simulink model "modello_Sabas_friend"  (R2020b)
settings: Solver=FixedStepAuto  StartTime=0.0  StopTime=5000  MinStep=0.009999  RelTol=1e-3
undefined symbols (not defined in the file or in its folder): Omega_0, omega_0
libraries: simulink x3, vrlib x1, aerolibatmos2 x1, sharedutil x1, aerolibgravity2 x1, sharedtransform x1
settings Model: Creator=Qmars  LastModifiedBy=Alessia

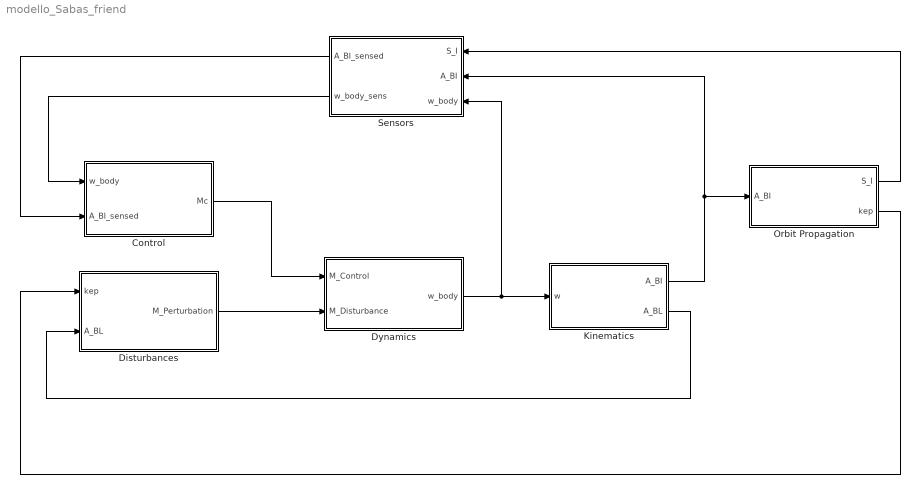
== system modello_Sabas_friend ==
  Control : Subsystem  mask{Control_Option=Target Pointing, MagMax=1.19, MagTorq_error=0.005, sample_rate_Mag=10, Irw=1e-5, maxRPM=8000, RPM_acc=5, sample_rate_RW=1, maxRPMrate=100, K_Det_x=-0.005*0.1585, K_Det_y=-0.005*0.0921, K_Det_z=-0.005*0.0866, Kp_Target_Pointing_x=-0.0027*0.1585, Kp_Target_Pointing_y=-0.0027*0.0921, Kp_Target_Pointing_z=-0.0027*0.0866, Kd_Target_Pointing_x=-0.104*0.1585, Kd_Target_Pointing_y=-0.104*0.0921, Kd_Target_Pointing_z=-0.104*0.0866}
      mask prompts: Control_Option "Choose your desired control strategy:"; MagMax "Max Magnetic Dipole (A.m^2)"; MagTorq_error "Dipole Error (A.m^2)"; sample_rate_Mag "Sample Rate [Hz]"; Irw "Moment of Inertia [kg.m^2]"; maxRPM "Max RPM"; RPM_acc "RPM Accuracy"; sample_rate_RW "Sample Rate [Hz]"; maxRPMrate "Max RPM Rate"
      mask TypeOptions Control_Option: No Control | Detumbling | Target Pointing
      mask DialogControl Container6 Prompt: Control Strategy
      mask DialogControl Container7 Prompt: Magnetorqure
      mask DialogControl Container8 Prompt: Reaction Wheels
      mask DialogControl Container10 Prompt: Detumbling Parameters
      mask DialogControl Container11 Prompt: Target Pointing
      mask Display: disp("Control")
  Disturbances : Subsystem  mask{rho_s_main=0.5, rho_d_main=0.1, rho_s_SP=0, rho_d_SP=0, C_D_main=2.2, C_D_SP=2.2}
      mask prompts: rho_s_main "Specular Reflection Coefficient"; rho_d_main "Diffusion Coefficient"; rho_s_SP "Specular Reflection Coefficient"; rho_d_SP "Diffusion Coefficient"; C_D_main "Drag Coefficient"; C_D_SP "Drag Coefficient"
      mask DialogControl Container4 Prompt: Radiation Constants
      mask DialogControl Container5 Prompt: Main Body
      mask DialogControl Container6 Prompt: Solar Panels
      mask DialogControl Container7 Prompt: Aerodynamics
      mask DialogControl Container10 Prompt: Main Body
      mask DialogControl Container11 Prompt: Solar Panels
      mask Display: disp("Disturbances")
  Dynamics : Subsystem  mask{m_main=9, b=0.1, d=0.3, a=0.2, m_SP=0.6, c=0.2, w_x_0=0.5, w_y_0=0.5, w_z_0=0.5}
      mask prompts: m_main "Mass [kg]"; b "Length in the X direction [m]"; d "Length in the Y direction [m]"; a "Length in the Z direction [m]"; m_SP "Mass [kg]"; c "Width in the Z direction [m]"; w_x_0 "Initial angular velocity in the X direction [deg/sec]"; w_y_0 "Initial angular velocity in the Y direction [deg/sec]"; w_z_0 "Initial angular velocity in the Z direction [deg/sec]"
      mask DialogControl Container4 Prompt: Satellite Characteristics
      mask DialogControl Container5 Prompt: Main Body
      mask DialogControl Container6 Prompt: Solar Panels
      mask DialogControl Container7 Prompt: Initial Conditions
      mask Display: disp("Dynamics")
  Kinematics : Subsystem  mask{theta_1_0=10, theta_2_0=10, theta_3_0=10}
      mask prompts: theta_1_0 "First Angle [deg]"; theta_2_0 "Second Angle [deg]"; theta_3_0 "Third Angle [deg]"
      mask DialogControl Container4 Prompt: Initial Conditions
      mask Display: disp("Kinematics")
  Orbit Propagation : Subsystem  mask{a_orbit=7092, e=0.0641568, i=98, omega=0, theta_0=270, Year=2021, Month=3, Day=21, Hour=12, Minute=0, Second=0}
      mask prompts: a_orbit "Semi-Major Axis [km]"; e "Eccentricity"; i "Inclination [deg]"; omega "Angular Position of the Perigee [deg]"; theta_0 "Initial Satellite Position [deg]"; Month "Month [number]"
      mask DialogControl Container4 Prompt: Orbit
      mask DialogControl Container5 Prompt: Time
      mask Display: disp("Orbit Propagation")
  Sensors : Subsystem  mask{accuracy_Sun=0.5, sample_rate_Sun=5, accuracy_EH=0.25, sample_rate_EH=1, accuracy_Star=1/360, sample_rate_Star=5, Mag_acc=1, sample_rate_Mag=10, ARW=0.2, RRW=0.3, sample_rate_Gyro=10}
      mask prompts: accuracy_Sun "Accuracy [deg]"; sample_rate_Sun "Sample Rate [Hz]"; accuracy_EH "Accuracy [deg]"; sample_rate_EH "Sample Rate [Hz]"; accuracy_Star "Accuracy [deg]"; sample_rate_Star "Sample Rate [Hz]"; Mag_acc "Accuracy [deg]"; sample_rate_Mag "Sample Rate [Hz]"; ARW "Angular Random Walk(ARW) [deg/hr^0.5]"; RRW "Rate Random Walk(RRW) [deg/hr^1.5]"; sample_rate_Gyro "Sample Rate [Hz]"
      mask DialogControl Container4 Prompt: Attitude Sensors
      mask DialogControl Container7 Prompt: Sun Sensor
      mask DialogControl Container9 Prompt: Earth Horizon Sensor
      mask DialogControl Container10 Prompt: Star Sensor
      mask DialogControl Container14 Prompt: Magnetometer
      mask DialogControl Container11 Prompt: Gyro
      mask Display: disp("Sensors")
  wires:
  Disturbances/1(M_Perturbation) -> Dynamics/2(M_Disturbance)
  Dynamics/1(w_body) -> Sensors/3(w_body), Kinematics/1(w)
  Kinematics/1(A_BI) -> Orbit Propagation/1(A_BI), Sensors/2(A_BI)
  Orbit Propagation/1(S_I) -> Sensors/1(S_I)
  Kinematics/2(A_BL) -> Disturbances/2(A_BL)
  Sensors/2(w_body_sens) -> Control/1(w_body)
  Control/1(Mc) -> Dynamics/1(M_Control)
  Sensors/1(A_BI_sensed) -> Control/2(A_BI_sensed)
  Orbit Propagation/2(kep) -> Disturbances/1(kep)

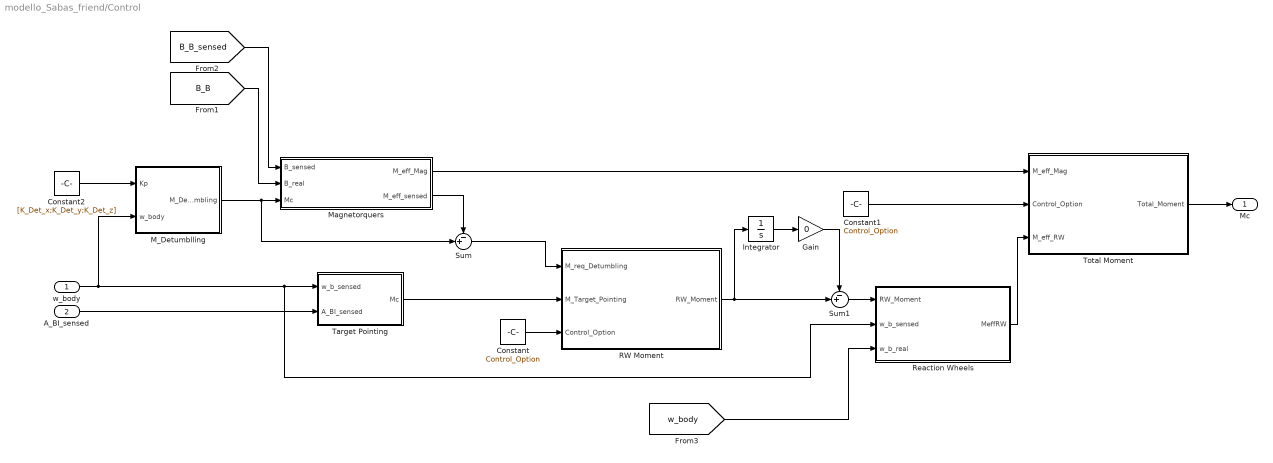
== system modello_Sabas_friend/Control ==
  w_body : Inport
  A_BI_sensed : Inport  Port=2
  Constant : Constant  Value=Control_Option
  Constant1 : Constant  Value=Control_Option
  Constant2 : Constant  Value=[K_Det_x;K_Det_y;K_Det_z]
  Gain : Gain  Gain=0
  Integrator : Integrator
  M_Detumblling : MATLAB Function  TreatAsAtomicUnit=on
  Magnetorquers : Subsystem
  RW Moment : MATLAB Function  TreatAsAtomicUnit=on
  Reaction Wheels : Subsystem
  Sum : Sum  Inputs=-+|
  Sum1 : Sum  Inputs=-+|
  Target Pointing : Subsystem
  Total Moment : MATLAB Function  TreatAsAtomicUnit=on
  Mc : Outport
  wires:
  M_Detumblling/1(M_Detumbling) -> Sum/2, Magnetorquers/3(Mc)
  w_body/1 -> M_Detumblling/2(w_body), Reaction Wheels/2(w_b_sensed), Target Pointing/1(w_b_sensed)
  A_BI_sensed/1 -> Target Pointing/2(A_BI_sensed)
  [B_B] -> Magnetorquers/2(B_real)
  [B_B_sensed] -> Magnetorquers/1(B_sensed)
  Target Pointing/1(Mc) -> RW Moment/2(M_Target_Pointing)
  Magnetorquers/2(M_eff_sensed) -> Sum/1
  Sum/1 -> RW Moment/1(M_req_Detumbling)
  Constant/1 -> RW Moment/3(Control_Option)
  RW Moment/1(RW_Moment) -> Integrator/1, Sum1/2
  [w_body] -> Reaction Wheels/3(w_b_real)
  Constant1/1 -> Total Moment/2(Control_Option)
  Reaction Wheels/1(MeffRW) -> Total Moment/3(M_eff_RW)
  Magnetorquers/1(M_eff_Mag) -> Total Moment/1(M_eff_Mag)
  Total Moment/1(Total_Moment) -> Mc/1
  Constant2/1 -> M_Detumblling/1(Kp)
  Sum1/1 -> Reaction Wheels/1(RW_Moment)
  Integrator/1 -> Gain/1
  Gain/1 -> Sum1/1

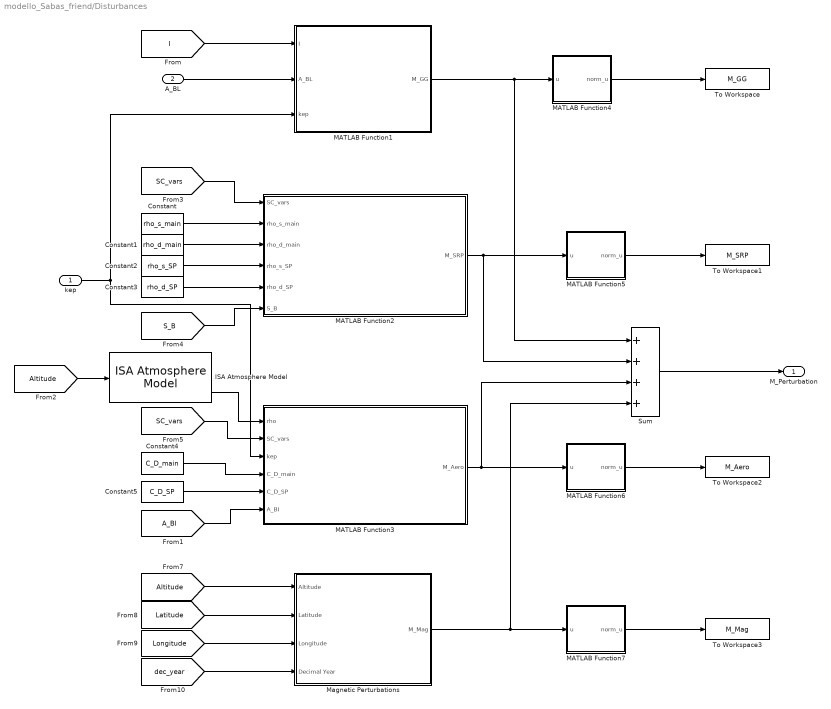
== system modello_Sabas_friend/Disturbances ==
  kep : Inport
  A_BL : Inport  Port=2
  Constant : Constant  Value=rho_s_main
  Constant1 : Constant  Value=rho_d_main
  Constant2 : Constant  Value=rho_s_SP
  Constant3 : Constant  Value=rho_d_SP
  Constant4 : Constant  Value=C_D_main
  Constant5 : Constant  Value=C_D_SP
  ISA Atmosphere Model : aerolibatmos2/ISA Atmosphere Model  custom=off  g=9.80665  gamma=1.4  R=287.0531  L=0.0065  h_trop=11000  h_strat=20000  rho0=1.225  P0=101325  T0=288.15  h0=0
  MATLAB Function1 : MATLAB Function  TreatAsAtomicUnit=on
  MATLAB Function2 : MATLAB Function  TreatAsAtomicUnit=on
  MATLAB Function3 : MATLAB Function  TreatAsAtomicUnit=on
  MATLAB Function4 : MATLAB Function  TreatAsAtomicUnit=on
  MATLAB Function5 : MATLAB Function  TreatAsAtomicUnit=on
  MATLAB Function6 : MATLAB Function  TreatAsAtomicUnit=on
  MATLAB Function7 : MATLAB Function  TreatAsAtomicUnit=on
  Magnetic Perturbations : Subsystem
  Sum : Sum  Inputs=++++
  To Workspace : ToWorkspace  VariableName=M_GG  SaveFormat=Structure With Time  SampleTime=-1
  To Workspace1 : ToWorkspace  VariableName=M_SRP  SaveFormat=Structure With Time  SampleTime=-1
  To Workspace2 : ToWorkspace  VariableName=M_Aero  SaveFormat=Structure With Time  SampleTime=-1
  To Workspace3 : ToWorkspace  VariableName=M_Mag  SaveFormat=Structure With Time  SampleTime=-1
  M_Perturbation : Outport
  wires:
  [dec_year] -> Magnetic Perturbations/4(Decimal Year)
  [I] -> MATLAB Function1/1(I)
  A_BL/1 -> MATLAB Function1/2(A_BL)
  [SC_vars] -> MATLAB Function2/1(SC_vars)
  Constant/1 -> MATLAB Function2/2(rho_s_main)
  [S_B] -> MATLAB Function2/6(S_B)
  Constant1/1 -> MATLAB Function2/3(rho_d_main)
  Constant2/1 -> MATLAB Function2/4(rho_s_SP)
  Constant3/1 -> MATLAB Function2/5(rho_d_SP)
  [SC_vars] -> MATLAB Function3/2(SC_vars)
  kep/1 -> MATLAB Function1/3(kep), MATLAB Function3/3(kep)
  Constant4/1 -> MATLAB Function3/4(C_D_main)
  Constant5/1 -> MATLAB Function3/5(C_D_SP)
  [Latitude] -> Magnetic Perturbations/2(Latitude)
  [Altitude] -> Magnetic Perturbations/1(Altitude)
  [Longitude] -> Magnetic Perturbations/3(Longitude)
  MATLAB Function1/1(M_GG) -> Sum/1, MATLAB Function4/1(u)
  MATLAB Function2/1(M_SRP) -> MATLAB Function5/1(u), Sum/2
  MATLAB Function3/1(M_Aero) -> MATLAB Function6/1(u), Sum/3
  Magnetic Perturbations/1(M_Mag) -> MATLAB Function7/1(u), Sum/4
  Sum/1 -> M_Perturbation/1
  [A_BI] -> MATLAB Function3/6(A_BI)
  ISA Atmosphere Model/4 -> MATLAB Function3/1(rho)
  [Altitude] -> ISA Atmosphere Model/1
  MATLAB Function4/1(norm_u) -> To Workspace/1
  MATLAB Function5/1(norm_u) -> To Workspace1/1
  MATLAB Function6/1(norm_u) -> To Workspace2/1
  MATLAB Function7/1(norm_u) -> To Workspace3/1

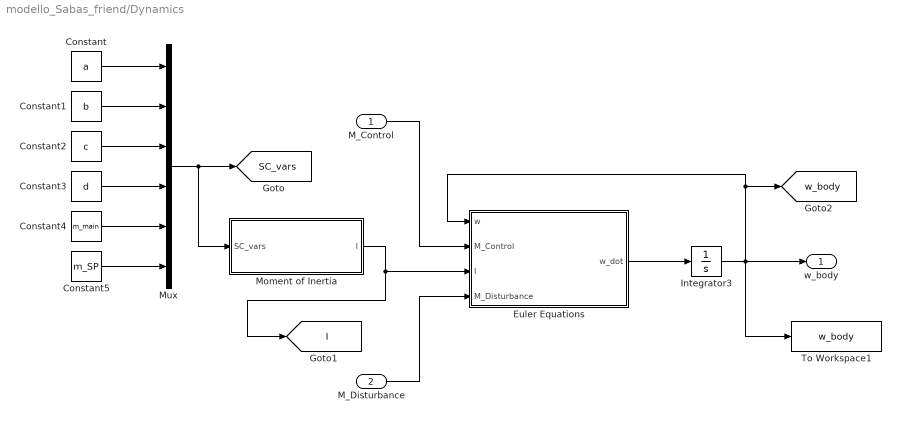
== system modello_Sabas_friend/Dynamics ==
  M_Control : Inport
  M_Disturbance : Inport  Port=2
  Constant : Constant  Value=a
  Constant1 : Constant  Value=b
  Constant2 : Constant  Value=c
  Constant3 : Constant  Value=d
  Constant4 : Constant  Value=m_main
  Constant5 : Constant  Value=m_SP
  Euler Equations : MATLAB Function  TreatAsAtomicUnit=on
  Integrator3 : Integrator  InitialCondition=pi*[w_x_0;w_y_0;w_z_0]/180
  Moment of Inertia : MATLAB Function  TreatAsAtomicUnit=on
  Mux : Mux  Inputs=6
  To Workspace1 : ToWorkspace  VariableName=w_body  SaveFormat=Timeseries  SampleTime=-1
  w_body : Outport
  tag scope: I=global, SC_vars=global, w_body=global
  wires:
  Integrator3/1 -> To Workspace1/1, w_body/1, Euler Equations/1(w), [w_body]
  Moment of Inertia/1(I) -> Euler Equations/3(I), [I]
  Euler Equations/1(w_dot) -> Integrator3/1
  M_Control/1 -> Euler Equations/2(M_Control)
  M_Disturbance/1 -> Euler Equations/4(M_Disturbance)
  Constant/1 -> Mux/1
  Constant1/1 -> Mux/2
  Constant2/1 -> Mux/3
  Constant3/1 -> Mux/4
  Constant4/1 -> Mux/5
  Constant5/1 -> Mux/6
  Mux/1 -> Moment of Inertia/1(SC_vars), [SC_vars]

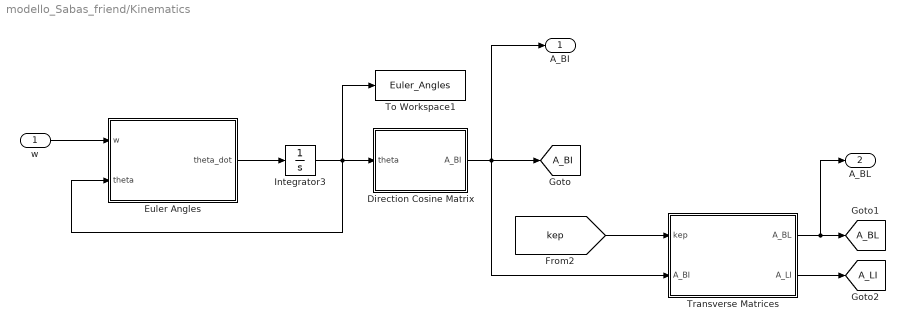
== system modello_Sabas_friend/Kinematics ==
  w : Inport
  Direction Cosine Matrix : MATLAB Function  TreatAsAtomicUnit=on
  Euler Angles : MATLAB Function  TreatAsAtomicUnit=on
  Integrator3 : Integrator  InitialCondition=pi*[theta_1_0;theta_2_0;theta_3_0]/180
  To Workspace1 : ToWorkspace  VariableName=Euler_Angles  SaveFormat=Timeseries  SampleTime=-1
  Transverse Matrices : MATLAB Function  TreatAsAtomicUnit=on
  A_BI : Outport
  A_BL : Outport  Port=2
  tag scope: A_BI=global, A_BL=global, A_LI=global
  wires:
  Integrator3/1 -> To Workspace1/1, Direction Cosine Matrix/1(theta), Euler Angles/2(theta)
  Euler Angles/1(theta_dot) -> Integrator3/1
  w/1 -> Euler Angles/1(w)
  Direction Cosine Matrix/1(A_BI) -> A_BI/1, Transverse Matrices/2(A_BI), [A_BI]
  Transverse Matrices/1(A_BL) -> [A_BL], A_BL/1
  [kep] -> Transverse Matrices/1(kep)
  Transverse Matrices/2(A_LI) -> [A_LI]

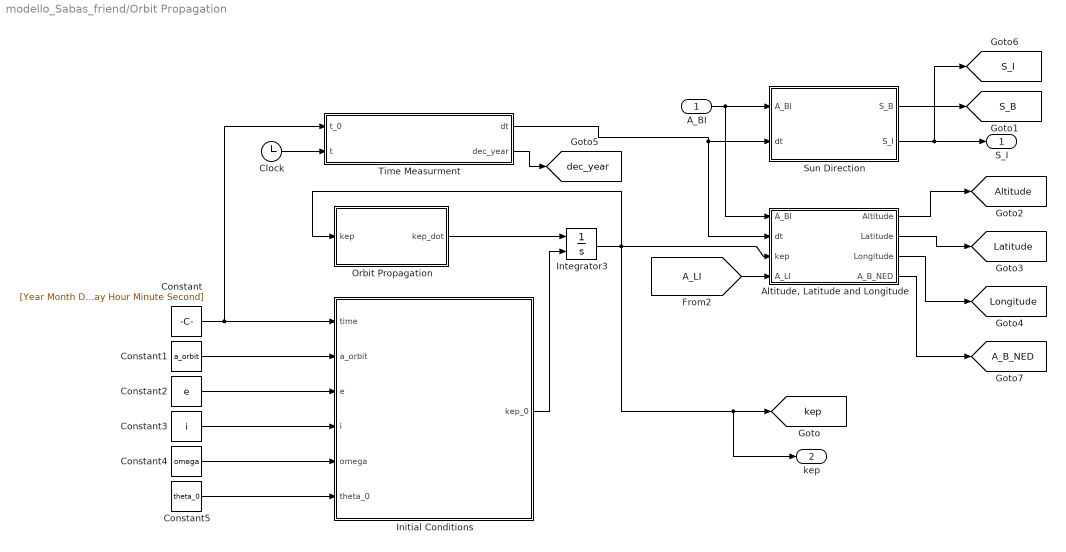
== system modello_Sabas_friend/Orbit Propagation ==
  A_BI : Inport
  "Altitude, Latitude and Longitude" : MATLAB Function  TreatAsAtomicUnit=on
  Clock : Clock
  Constant : Constant  Value=[Year Month Day Hour Minute Second]
  Constant1 : Constant  Value=a_orbit
  Constant2 : Constant  Value=e
  Constant3 : Constant  Value=i
  Constant4 : Constant  Value=omega
  Constant5 : Constant  Value=theta_0
  Initial Conditions : MATLAB Function  TreatAsAtomicUnit=on
  Integrator3 : Integrator  InitialConditionSource=external  InitialCondition=[a_orbit;e;i;Omega_0;omega_0;theta_0]
  Orbit Propagation : MATLAB Function  TreatAsAtomicUnit=on
  Sun Direction : MATLAB Function  TreatAsAtomicUnit=on
  Time Measurment : MATLAB Function  TreatAsAtomicUnit=on
  S_I : Outport
  kep : Outport  Port=2
  tag scope: A_B_NED=global, Altitude=global, Latitude=global, Longitude=global, S_B=global, S_I=global, dec_year=global, kep=global
  wires:
  Orbit Propagation/1(kep_dot) -> Integrator3/1
  Integrator3/1 -> Orbit Propagation/1(kep), "Altitude, Latitude and Longitude"/3(kep), kep/1, [kep]
  A_BI/1 -> "Altitude, Latitude and Longitude"/1(A_BI), Sun Direction/1(A_BI)
  Sun Direction/2(S_I) -> [S_I], S_I/1
  Sun Direction/1(S_B) -> [S_B]
  Initial Conditions/1(kep_0) -> Integrator3/2
  Constant/1 -> Initial Conditions/1(time), Time Measurment/1(t_0)
  Constant1/1 -> Initial Conditions/2(a_orbit)
  Constant2/1 -> Initial Conditions/3(e)
  Constant5/1 -> Initial Conditions/6(theta_0)
  Constant4/1 -> Initial Conditions/5(omega)
  Constant3/1 -> Initial Conditions/4(i)
  Clock/1 -> Time Measurment/2(t)
  Time Measurment/1(dt) -> "Altitude, Latitude and Longitude"/2(dt), Sun Direction/2(dt)
  "Altitude, Latitude and Longitude"/1(Altitude) -> [Altitude]
  "Altitude, Latitude and Longitude"/3(Longitude) -> [Longitude]
  "Altitude, Latitude and Longitude"/2(Latitude) -> [Latitude]
  [A_LI] -> "Altitude, Latitude and Longitude"/4(A_LI)
  Time Measurment/2(dec_year) -> [dec_year]
  "Altitude, Latitude and Longitude"/4(A_B_NED) -> [A_B_NED]

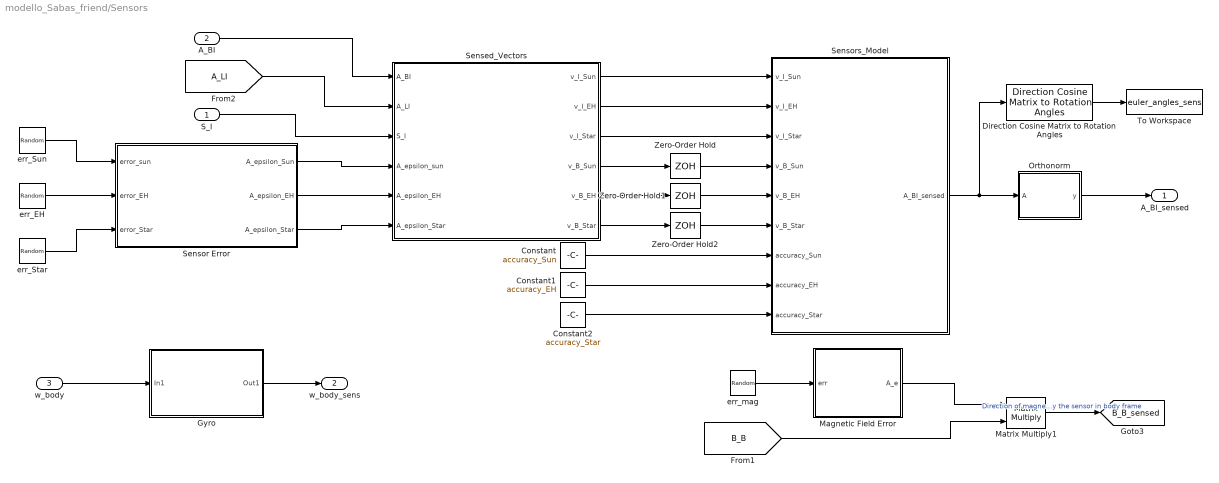
== system modello_Sabas_friend/Sensors ==
  S_I : Inport
  A_BI : Inport  Port=2
  w_body : Inport  Port=3
  Constant : Constant  Value=accuracy_Sun
  Constant1 : Constant  Value=accuracy_EH
  Constant2 : Constant  Value=accuracy_Star
  Direction Cosine Matrix to Rotation Angles : sharedtransform/Direction Cosine Matrix to Rotation Angles  rotationOrder=ZYX  aMode=aMode  action=None  tolerance=eps(2)
      settings: SourceProductBaseCode=AE,PW,DR,MT,UV,VE
  Gyro : Subsystem
  Magnetic Field Error : MATLAB Function  TreatAsAtomicUnit=on
  Matrix Multiply1 : Product  Multiplication=Matrix(*)
  Orthonorm : MATLAB Function  TreatAsAtomicUnit=on
  Sensed_Vectors : MATLAB Function  TreatAsAtomicUnit=on
  Sensor Error : MATLAB Function  TreatAsAtomicUnit=on
  Sensors_Model : MATLAB Function  TreatAsAtomicUnit=on
  To Workspace : ToWorkspace  VariableName=euler_angles_sens  SaveFormat=Timeseries  SampleTime=-1
  Zero-Order Hold : ZeroOrderHold  SampleTime=1/sample_rate_Sun
  Zero-Order Hold1 : ZeroOrderHold  SampleTime=1/sample_rate_EH
  Zero-Order Hold2 : ZeroOrderHold  SampleTime=1/sample_rate_Star
  err_EH : RandomNumber  Variance=(1/4*deg2rad(accuracy_EH*[1 1 1])).^2  Seed=[4 5 6]  SampleTime=1/10
  err_Star : RandomNumber  Variance=(1/4*deg2rad(accuracy_Star*[1 1 1])).^2  Seed=[4 5 6]  SampleTime=1/10
  err_Sun : RandomNumber  Variance=(1/4*deg2rad(accuracy_Sun*[1 1 1])).^2  Seed=[1 2 3]  SampleTime=1/10
  err_mag : RandomNumber  Variance=(1/4*deg2rad(Mag_acc*[1;1;1])).^2  Seed=[1 2 3]  SampleTime=1/sample_rate_Mag
  A_BI_sensed : Outport
  w_body_sens : Outport  Port=2
  tag scope: B_B_sensed=global
  wires:
  err_Sun/1 -> Sensor Error/1(error_sun)
  Constant1/1 -> Sensors_Model/8(accuracy_EH)
  S_I/1 -> Sensed_Vectors/3(S_I)
  err_Star/1 -> Sensor Error/3(error_Star)
  err_EH/1 -> Sensor Error/2(error_EH)
  A_BI/1 -> Sensed_Vectors/1(A_BI)
  Sensors_Model/1(A_BI_sensed) -> Direction Cosine Matrix to Rotation Angles/1, Orthonorm/1(A)
  [A_LI] -> Sensed_Vectors/2(A_LI)
  Constant/1 -> Sensors_Model/7(accuracy_Sun)
  Constant2/1 -> Sensors_Model/9(accuracy_Star)
  Orthonorm/1(y) -> A_BI_sensed/1
  Sensor Error/1(A_epsilon_Sun) -> Sensed_Vectors/4(A_epsilon_sun)
  Sensor Error/2(A_epsilon_EH) -> Sensed_Vectors/5(A_epsilon_EH)
  Sensor Error/3(A_epsilon_Star) -> Sensed_Vectors/6(A_epsilon_Star)
  Sensed_Vectors/2(v_I_EH) -> Sensors_Model/2(v_I_EH)
  Sensed_Vectors/3(v_I_Star) -> Sensors_Model/3(v_I_Star)
  Sensed_Vectors/4(v_B_Sun) -> Zero-Order Hold/1
  Sensed_Vectors/5(v_B_EH) -> Zero-Order Hold1/1
  Sensed_Vectors/6(v_B_Star) -> Zero-Order Hold2/1
  Sensed_Vectors/1(v_I_Sun) -> Sensors_Model/1(v_I_Sun)
  Zero-Order Hold/1 -> Sensors_Model/4(v_B_Sun)
  Zero-Order Hold1/1 -> Sensors_Model/5(v_B_EH)
  Zero-Order Hold2/1 -> Sensors_Model/6(v_B_Star)
  Direction Cosine Matrix to Rotation Angles/1 -> To Workspace/1
  w_body/1 -> Gyro/1(In1)
  Gyro/1(Out1) -> w_body_sens/1
  err_mag/1 -> Magnetic Field Error/1(err)
  Magnetic Field Error/1(A_e) -> Matrix Multiply1/1
  [B_B] -> Matrix Multiply1/2
  Matrix Multiply1/1 -> [B_B_sensed]  "Direction of magnetic field vector determined by the sensor in body frame"

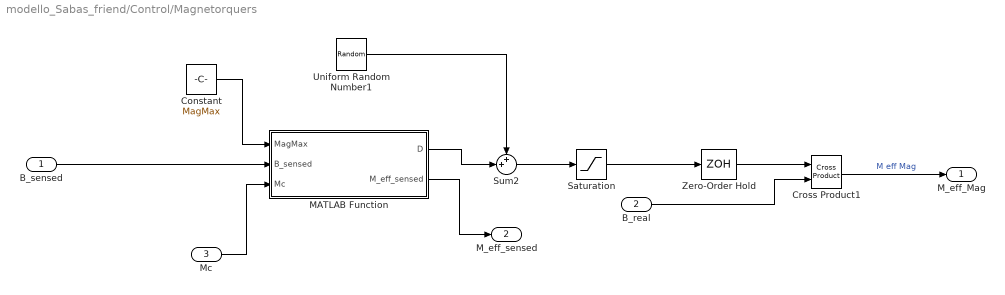
== system modello_Sabas_friend/Control/Magnetorquers ==
  B_sensed : Inport
  B_real : Inport  Port=2
  Mc : Inport  Port=3
  Constant : Constant  Value=MagMax
  Cross Product1 : vrlib/Utilities/Cross Product
  MATLAB Function : MATLAB Function  TreatAsAtomicUnit=on
  Saturation : Saturate  UpperLimit=MagMax  LowerLimit=-MagMax
  Sum2 : Sum  Inputs=++|
  Uniform Random Number1 : UniformRandomNumber  Minimum=-MagTorq_error*[1;1;1]  Maximum=MagTorq_error*[1;1;1]  Seed=456156  SampleTime=1/sample_rate_Mag
  Zero-Order Hold : ZeroOrderHold  SampleTime=1/sample_rate_Mag
  M_eff_Mag : Outport
  M_eff_sensed : Outport  Port=2
  wires:
  B_sensed/1 -> MATLAB Function/2(B_sensed)
  Saturation/1 -> Zero-Order Hold/1
  Cross Product1/1 -> M_eff_Mag/1  "M eff Mag"
  Sum2/1 -> Saturation/1
  Zero-Order Hold/1 -> Cross Product1/1
  Constant/1 -> MATLAB Function/1(MagMax)
  MATLAB Function/1(D) -> Sum2/2
  B_real/1 -> Cross Product1/2
  Mc/1 -> MATLAB Function/3(Mc)
  Uniform Random Number1/1 -> Sum2/1
  MATLAB Function/2(M_eff_sensed) -> M_eff_sensed/1

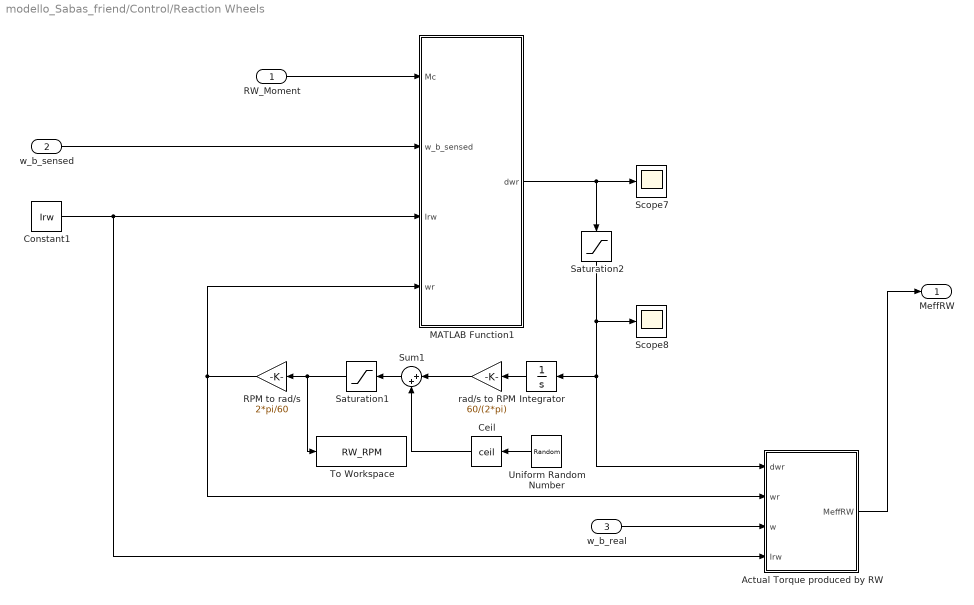
== system modello_Sabas_friend/Control/Reaction Wheels ==
  RW_Moment : Inport
  w_b_sensed : Inport  Port=2
  w_b_real : Inport  Port=3
  Actual Torque produced by RW : MATLAB Function  TreatAsAtomicUnit=on
  Ceil : Rounding  Operator=ceil
  Constant1 : Constant  Value=Irw
  Integrator : Integrator  InitialCondition=[0;0;0]
  MATLAB Function1 : MATLAB Function  TreatAsAtomicUnit=on
  RPM to rad/s : Gain  Gain=2*pi/60
  Saturation1 : Saturate  UpperLimit=maxRPM*[1;1;1]  LowerLimit=-maxRPM*[1;1;1]  LinearizeAsGain=off  ZeroCross=off
  Saturation2 : Saturate  UpperLimit=maxRPMrate  LowerLimit=-maxRPMrate
  Scope7 : Scope
  Scope8 : Scope
  Sum1 : Sum  Inputs=|++
  To Workspace : ToWorkspace  VariableName=RW_RPM  SaveFormat=Structure With Time  SampleTime=-1
  Uniform Random Number : UniformRandomNumber  Minimum=-RPM_acc*[1;1;1]  Maximum=RPM_acc*[1;1;1]  Seed=561651  SampleTime=1/sample_rate_RW
  rad/s to RPM : Gain  Gain=60/(2*pi)
  MeffRW : Outport
  wires:
  Ceil/1 -> Sum1/2
  rad/s to RPM/1 -> Sum1/1
  RPM to rad/s/1 -> MATLAB Function1/4(wr), Actual Torque produced by RW/2(wr)
  Constant1/1 -> Actual Torque produced by RW/4(Irw), MATLAB Function1/3(Irw)
  w_b_real/1 -> Actual Torque produced by RW/3(w)
  MATLAB Function1/1(dwr) -> Saturation2/1, Scope7/1
  Integrator/1 -> rad/s to RPM/1
  Saturation1/1 -> To Workspace/1, RPM to rad/s/1
  Uniform Random Number/1 -> Ceil/1
  Sum1/1 -> Saturation1/1
  w_b_sensed/1 -> MATLAB Function1/2(w_b_sensed)
  Actual Torque produced by RW/1(MeffRW) -> MeffRW/1
  RW_Moment/1 -> MATLAB Function1/1(Mc)
  Saturation2/1 -> Actual Torque produced by RW/1(dwr), Integrator/1, Scope8/1

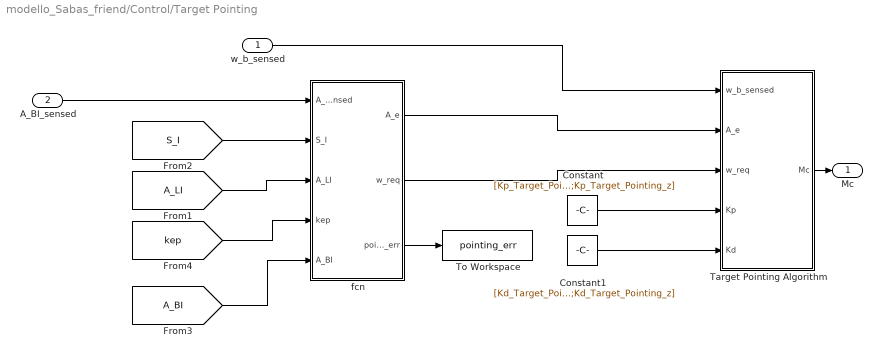
== system modello_Sabas_friend/Control/Target Pointing ==
  w_b_sensed : Inport
  A_BI_sensed : Inport  Port=2
  Constant : Constant  Value=[Kp_Target_Pointing_x;Kp_Target_Pointing_y;Kp_Target_Pointing_z]
  Constant1 : Constant  Value=[Kd_Target_Pointing_x;Kd_Target_Pointing_y;Kd_Target_Pointing_z]
  Target Pointing Algorithm : MATLAB Function  TreatAsAtomicUnit=on
  To Workspace : ToWorkspace  VariableName=pointing_err  SaveFormat=Timeseries  SampleTime=-1
  fcn : MATLAB Function  TreatAsAtomicUnit=on
  Mc : Outport
  wires:
  fcn/3(pointing_err) -> To Workspace/1
  [kep] -> fcn/4(kep)
  fcn/2(w_req) -> Target Pointing Algorithm/3(w_req)
  Constant1/1 -> Target Pointing Algorithm/5(Kd)
  [S_I] -> fcn/2(S_I)
  [A_BI] -> fcn/5(A_BI)
  [A_LI] -> fcn/3(A_LI)
  fcn/1(A_e) -> Target Pointing Algorithm/2(A_e)
  Constant/1 -> Target Pointing Algorithm/4(Kp)
  A_BI_sensed/1 -> fcn/1(A_BI_sensed)
  Target Pointing Algorithm/1(Mc) -> Mc/1
  w_b_sensed/1 -> Target Pointing Algorithm/1(w_b_sensed)

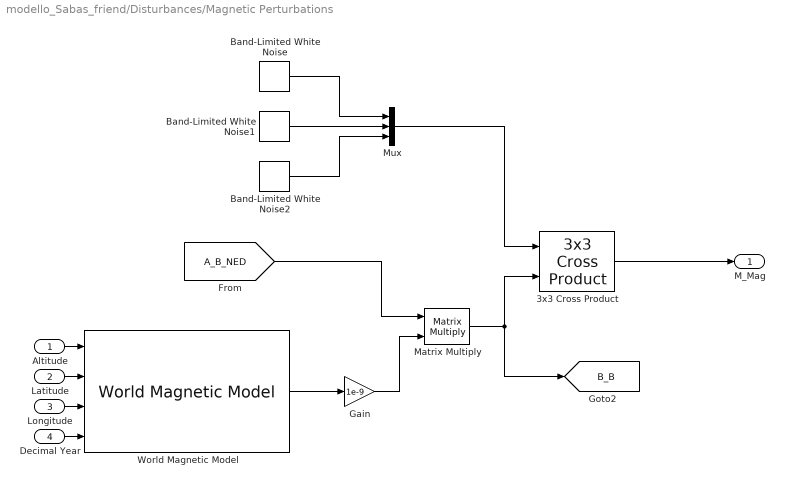
== system modello_Sabas_friend/Disturbances/Magnetic Perturbations ==
  Altitude : Inport
  Latitude : Inport  Port=2
  Longitude : Inport  Port=3
  Decimal Year : Inport  Port=4
  3x3 Cross Product : sharedutil/3x3 Cross Product  aMode=aMode
      settings: SourceProductBaseCode=AE,PW,DR,MT,UV,VE
  Band-Limited White Noise : simulink/Sources/Band-Limited White Noise  Cov=[0.1]  Ts=0.1  seed=[23341]
  Band-Limited White Noise1 : simulink/Sources/Band-Limited White Noise  Cov=[0.1]  Ts=0.1  seed=[23341]
  Band-Limited White Noise2 : simulink/Sources/Band-Limited White Noise  Cov=[0.1]  Ts=0.1  seed=[23341]
  Gain : Gain  Gain=1e-9
  Matrix Multiply : Product  Multiplication=Matrix(*)
  Mux : Mux  Inputs=3
  World Magnetic Model : aerolibgravity2/World Magnetic Model  model=Custom  customFile='WMM2020.COF'  units=Metric (MKS)  time_in=on  month=January  day=1  year=2020  action=None  h_out=off  dec_out=off  inc_out=off  ti_out=off
      settings: SourceProductBaseCode=AE
  M_Mag : Outport
  tag scope: B_B=global
  wires:
  World Magnetic Model/1 -> Gain/1
  Band-Limited White Noise/1 -> Mux/1
  Latitude/1 -> World Magnetic Model/2
  Band-Limited White Noise1/1 -> Mux/2
  Altitude/1 -> World Magnetic Model/1
  Band-Limited White Noise2/1 -> Mux/3
  Matrix Multiply/1 -> [B_B], 3x3 Cross Product/2
  Mux/1 -> 3x3 Cross Product/1
  [A_B_NED] -> Matrix Multiply/1
  Decimal Year/1 -> World Magnetic Model/4
  3x3 Cross Product/1 -> M_Mag/1
  Longitude/1 -> World Magnetic Model/3
  Gain/1 -> Matrix Multiply/2

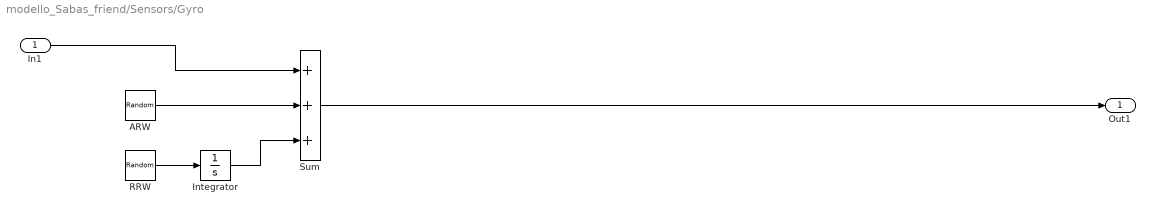
== system modello_Sabas_friend/Sensors/Gyro ==
  In1 : Inport
  ARW : RandomNumber  Variance=(1/4*deg2rad(ARW*[1;1;1]/sqrt(3600))).^2  Seed=1  SampleTime=1/sample_rate_Gyro
  Integrator : Integrator
  RRW : RandomNumber  Variance=(1/4*deg2rad(RRW*[1;1;1]/3600^3)).^2  Seed=2  SampleTime=1/sample_rate_Gyro
  Sum : Sum  Inputs=+++
  Out1 : Outport
  wires:
  Integrator/1 -> Sum/3
  ARW/1 -> Sum/2
  Sum/1 -> Out1/1
  RRW/1 -> Integrator/1
  In1/1 -> Sum/1

== matlab function modello_Sabas_friend/Orbit Propagation/Initial Conditions ==
  data: time input; a_orbit input; kep_0 output; e input; i input; omega input; theta_0 input
function kep_0  = Initial_Kepler_Elements(time, a_orbit, e, i, omega, theta_0)

R_s = 149597870.691; % 1AU [km]
mu_s = 132712440017.987;
n_s  = sqrt(mu_s/R_s^3);

t_initial = datetime(time(1),time(2),time(3),time(4),time(5),time(6));
t_spring = datetime(time(1),3,21,12,0,0);

t = seconds(t_initial - t_spring);
kep_0 = zeros(6,1);
kep_0(1,1) = a_orbit;
kep_0(2,1) = e;
kep_0(3,1) = deg2rad(i);
kep_0(4,1) = n_s*t;
kep_0(5,1) = deg2rad(omega);
kep_0(6,1) = deg2rad(theta_0);

== matlab function modello_Sabas_friend/Disturbances/MATLAB Function1 ==
  data: I input; M_GG output; A_BL input; kep input
function M_GG = gravity_gradient_torque(I, A_BL, kep)

G = 6.67408e-11;
m_E = 5.972e+24;
a  = kep(1);
e  = kep(2);
th = kep(6);
p = a*(1-e^2);
R = p / (1+e*cos(th)) * 1e+3; % [m]

% Moments of Inertia [kg*m^2]
I1 = I(1,1);
I2 = I(2,2);
I3 = I(3,3);

C1 = (I2-I3)/I1;
C2 = (I3-I1)/I2;
C3 = (I1-I2)/I3;

%% Gravity Gradient Torque
c = A_BL * [1;0;0];

M_GG = [- 3*G*m_E/R^3 *C1* c(3)*c(2);
        - 3*G*m_E/R^3 *C2* c(1)*c(3);
        - 3*G*m_E/R^3 *C3* c(2)*c(1)];

== matlab function modello_Sabas_friend/Orbit Propagation/Time Measurment ==
  data: t_0 input; dt output; t input; dec_year output
function [dt, dec_year]  = time_measurment(t_0, t)

t_now = datetime(t_0(1),t_0(2),t_0(3),t_0(4),t_0(5),t_0(6)+t);
t_start_year = datetime(t_0(1),0,0,0,0,0);
t_end_year = datetime(t_0(1)+1,0,0,0,0,0);
t_spring = datetime(t_0(1),3,21,12,0,0);

dt = seconds(t_now - t_spring);
dt_1 = seconds(t_now-t_start_year);
dt_2 = seconds(t_end_year - t_start_year);
dec_year = t_0(1)+dt_1/dt_2;

== matlab function modello_Sabas_friend/Orbit Propagation/Altitude, Latitude and Longitude ==
  data: A_BI input; dt input; Altitude output; Latitude output; kep input; Longitude output; A_LI input; A_B_NED output
function [Altitude, Latitude, Longitude, A_B_NED] = fcn(A_BI, dt, kep, A_LI)


a  = kep(1);
e  = kep(2);
th = kep(6);
p = a*(1-e^2); % [km]
R = p / (1+e*cos(th)) * 1e+3; % [m]

R_I = A_LI'*[R;0;0];
Altitude = R - 6371000;
delta = asin(R_I(3,1)/R); % declination [rad]
if R_I(2,1)>0
    alpha = acos(R_I(1,1)/sqrt(R_I(1,1)^2+R_I(2,1)^2));
else
    alpha = pi - acos(R_I(1,1)/sqrt(R_I(1,1)^2+R_I(2,1)^2));
end

w_E = 2*pi/(23*3600 + 56*60 + 4.09);
Latitude = rad2deg(delta);
Longitude = rad2deg(alpha - w_E*dt);

A_NED_I = [cos(delta),0,+sin(pi/2+delta);0,1,0;-sin(pi/2+delta),0,cos(delta)]*[cos(alpha),sin(alpha),0;-sin(alpha),cos(alpha),0;0,0,1];
A_B_NED = A_BI*A_NED_I';

== matlab function modello_Sabas_friend/Sensors/Sensor Error ==
  data: error_sun input; A_epsilon_Sun output; error_EH input; A_epsilon_EH output; error_Star input; A_epsilon_Star output
function [A_epsilon_Sun, A_epsilon_EH, A_epsilon_Star] = sensor_error(error_sun, error_EH, error_Star)

%% Sun Sensor
psi_acc = error_sun(1);
th_acc  = error_sun(2);
phi_acc = error_sun(3);
A_epsilon_Sun = [cos(psi_acc)*cos(th_acc)  (cos(psi_acc)*sin(th_acc)*sin(phi_acc)+sin(psi_acc)*cos(phi_acc)) (-cos(psi_acc)*sin(th_acc)*cos(phi_acc)+sin(psi_acc)*sin(phi_acc));
                -sin(psi_acc)*cos(th_acc) (-sin(psi_acc)*sin(th_acc)*sin(phi_acc)+cos(psi_acc)*cos(phi_acc))  (sin(psi_acc)*sin(th_acc)*cos(phi_acc)+cos(psi_acc)*sin(phi_acc));
                 sin(th_acc)               -cos(th_acc)*sin(phi_acc)                                           cos(th_acc)*cos(phi_acc)];

%% Earth Horizon Sensor
psi_acc = error_EH(1);
th_acc  = error_EH(2);
phi_acc = error_EH(3);
A_epsilon_EH = [cos(psi_acc)*cos(th_acc)  (cos(psi_acc)*sin(th_acc)*sin(phi_acc)+sin(psi_acc)*cos(phi_acc)) (-cos(psi_acc)*sin(th_acc)*cos(phi_acc)+sin(psi_acc)*sin(phi_acc));
                -sin(psi_acc)*cos(th_acc) (-sin(psi_acc)*sin(th_acc)*sin(phi_acc)+cos(psi_acc)*cos(phi_acc))  (sin(psi_acc)*sin(th_acc)*cos(phi_acc)+cos(psi_acc)*sin(phi_acc));
                 sin(th_acc)               -cos(th_acc)*sin(phi_acc)                                           cos(th_acc)*cos(phi_acc)];

%% Star Sensor
psi_acc = error_Star(1);
th_acc  = error_Star(2);
phi_acc = error_Star(3);
A_epsilon_Star = [cos(psi_acc)*cos(th_acc)  (cos(psi_acc)*sin(th_acc)*sin(phi_acc)+sin(psi_acc)*cos(phi_acc)) (-cos(psi_acc)*sin(th_acc)*cos(phi_acc)+sin(psi_acc)*sin(phi_acc));
                -sin(psi_acc)*cos(th_acc) (-sin(psi_acc)*sin(th_acc)*sin(phi_acc)+cos(psi_acc)*cos(phi_acc))  (sin(psi_acc)*sin(th_acc)*cos(phi_acc)+cos(psi_acc)*sin(phi_acc));
                 sin(th_acc)               -cos(th_acc)*sin(phi_acc)                                           cos(th_acc)*cos(phi_acc)];


end

== matlab function modello_Sabas_friend/Sensors/Sensors_Model ==
  data: v_I_Sun input; v_I_EH input; v_I_Star input; v_B_Sun input; v_B_EH input; v_B_Star input; A_BI_sensed output; accuracy_Sun input; accuracy_EH input; accuracy_Star input
function A_BI_sensed = Sensors_Model(v_I_Sun, v_I_EH, v_I_Star, v_B_Sun, v_B_EH, v_B_Star, accuracy_Sun, accuracy_EH, accuracy_Star)

%% SVD algorithm for attitude estimation
prec_Sun = 1/norm(accuracy_Sun);
prec_EH = 1/norm(accuracy_EH);
prec_Star = 1/norm(accuracy_Star);
alpha = [prec_Sun prec_EH prec_Star] / (prec_Sun+prec_EH+prec_Star);


B = alpha(1)*v_B_Sun*v_I_Sun' + alpha(2)*v_B_EH*v_I_EH' + alpha(3)*v_B_Star*v_I_Star';

[U,~,V] = svd(B);
M = diag([1, 1, det(U)*det(V)]);
A_BI_sensed = U*M*V';

== matlab function modello_Sabas_friend/Sensors/Orthonorm ==
  data: A input; y output
function y = orthonorm(A)

% Recall: for a matrix to be orthonormal it is necessary that
%         det(A)=1  -->  tr(A'A - I) = 0

tol = 1e-7;
k = 0;
while trace(A'*A - eye(3,3)) > tol
    k = k+1;
    A = 3/2 * A - 1/2 * A*A'*A;
end

y = A;

== matlab function modello_Sabas_friend/Sensors/Sensed_Vectors ==
  data: A_BI input; A_LI input; v_I_Sun output; S_I input; A_epsilon_sun input; A_epsilon_EH input; A_epsilon_Star input; v_I_EH output; v_I_Star output; v_B_Sun output; v_B_EH output; v_B_Star output
function [v_I_Sun, v_I_EH, v_I_Star, v_B_Sun, v_B_EH, v_B_Star] = Sensed_Vectors(A_BI, A_LI, S_I, A_epsilon_sun, A_epsilon_EH, A_epsilon_Star)

E_I = -A_LI'*[1;0;0];
S_I = S_I / norm(S_I);
Polaris_I = [cosd(37.9545)*cosd(89.2641);sind(37.9545)*cosd(89.2641);sind(89.2641)];

v_I_Sun = S_I;
v_I_EH = E_I;
v_I_Star = Polaris_I;

v_B_Sun = A_epsilon_sun * A_BI * v_I_Sun;
v_B_EH = A_epsilon_EH * A_BI * v_I_EH;
v_B_Star = A_epsilon_Star * A_BI * v_I_Star;

== matlab function modello_Sabas_friend/Control/Target Pointing/fcn ==
  data: A_BI_sensed input; S_I input; A_LI input; kep input; A_BI input; A_e output; w_req output; pointing_err output
function [A_e, w_req, pointing_err]  = fcn(A_BI_sensed, S_I, A_LI, kep, A_BI)

%% Calculating Target Attitude Matrix
Z_B  = A_LI'*[-1;0;0];
sun_direction = S_I/norm(S_I);
X_B = sun_direction - dot(sun_direction,Z_B)*Z_B;
Y_B = cross(Z_B,X_B);

A_T = [X_B';Y_B';Z_B'];
A_e = A_BI_sensed*A_T';

%% Pointing Accuracy
Z_B_actual = A_BI'*[0;0;1];
pointing_err = rad2deg(acos(dot(Z_B,Z_B_actual)));

%% Calculating Target Angular Velocity
% kep = [a e i om, Om, th]
a  = kep(1);
e  = kep(2);
th = kep(6);

% Calculating orbital angular velocity
mu_e = 398600.433; % [km^3/s^2]
n_e = sqrt(mu_e/a^3);

w_req = A_BI_sensed*A_LI'*[0;0;n_e*(1+e*cos(th))^2 / ((1-e^2)^1.5)];

== matlab function modello_Sabas_friend/Control/Magnetorquers/MATLAB Function ==
  data: MagMax input; B_sensed input; Mc input; D output; M_eff_sensed output
function [D, M_eff_sensed] = fcn(MagMax,B_sensed,Mc)
D=1/dot(B_sensed,B_sensed)*cross(B_sensed,Mc);
if D(1)>MagMax
    D(1)=MagMax;
end
if D(2)>MagMax
    D(2)=MagMax;
end
if D(3)>MagMax
    D(3)=MagMax;
end
M_eff_sensed=cross(D,B_sensed);

== matlab function modello_Sabas_friend/Sensors/Magnetic Field Error ==
  data: err input; A_e output
function A_e = Mag_err(err)

%% Magentic Field Direction Error
psi_acc = err(1);
th_acc  = err(2);
phi_acc = err(3);
A_e = [cos(psi_acc)*cos(th_acc)  (cos(psi_acc)*sin(th_acc)*sin(phi_acc)+sin(psi_acc)*cos(phi_acc)) (-cos(psi_acc)*sin(th_acc)*cos(phi_acc)+sin(psi_acc)*sin(phi_acc));
                -sin(psi_acc)*cos(th_acc) (-sin(psi_acc)*sin(th_acc)*sin(phi_acc)+cos(psi_acc)*cos(phi_acc))  (sin(psi_acc)*sin(th_acc)*cos(phi_acc)+cos(psi_acc)*sin(phi_acc));
                 sin(th_acc)               -cos(th_acc)*sin(phi_acc)                                           cos(th_acc)*cos(phi_acc)];

end

== matlab function modello_Sabas_friend/Control/RW Moment ==
  data: M_req_Detumbling input; RW_Moment output; M_Target_Pointing input; Control_Option input
function RW_Moment = fcn(M_req_Detumbling, M_Target_Pointing, Control_Option)

if Control_Option == 0
    RW_Moment = [0;0;0];
elseif Control_Option == 1
    RW_Moment = M_req_Detumbling;
else
    RW_Moment = M_Target_Pointing;
end

== matlab function modello_Sabas_friend/Control/Reaction Wheels/Actual Torque produced by RW ==
  data: dwr input; MeffRW output; wr input; w input; Irw input
function MeffRW = fcn(dwr,wr,w,Irw)

A=[1 0 0; 0 1 0; 0 0 1];
Irw=Irw*eye(3);
hr=Irw*wr;
dhr=Irw*dwr;
MeffRW=-A*dhr-cross(w,A*hr);

== matlab function modello_Sabas_friend/Control/Reaction Wheels/MATLAB Function1 ==
  data: Mc input; w_b_sensed input; dwr output; Irw input; wr input
function dwr = fcn(Mc,w_b_sensed,Irw,wr)

A=[1 0 0; 0 1 0; 0 0 1];
Irwmat=Irw*eye(3);
hr=Irwmat*wr;
F=cross(A*hr,w_b_sensed)-Mc;
G=A\F;
dhr=G(1:3,1);
dwr=dhr/Irw;

== matlab function modello_Sabas_friend/Control/Total Moment ==
  data: M_eff_Mag input; Control_Option input; Total_Moment output; M_eff_RW input
function Total_Moment = fcn(M_eff_Mag, Control_Option, M_eff_RW)

if Control_Option == 1
    Total_Moment = [0;0;0];
elseif Control_Option == 2
    Total_Moment = M_eff_Mag + M_eff_RW;
else
    Total_Moment = M_eff_RW;
end

== matlab function modello_Sabas_friend/Disturbances/MATLAB Function2 ==
  data: SC_vars input; rho_s_main input; rho_d_main input; rho_s_SP input; rho_d_SP input; M_SRP output; S_B input
function M_SRP = sun_radiation_perturbation(SC_vars,rho_s_main,rho_d_main,rho_s_SP,rho_d_SP, S_B)

%% Satellite Characteristics
a = SC_vars(1,1);
b = SC_vars(2,1);
c = SC_vars(3,1);
d = SC_vars(4,1);
m_main = SC_vars(5,1);
m_SP = SC_vars(6,1);
%% SRP Torque
F_e = 1358 + 580 + 143.4;
P = F_e / (3*1e+8);

N_main = 6; % # main body surfaces
N_SP = 4; % # solar panel surfaces

N = zeros(N_main+N_SP,3);
A = zeros(N_main+N_SP,1);
r = zeros(N_main+N_SP,3);
n1 = [1 0 0];  n2 = [0 1 0];  n3 = [0 0 1];
% S/C Main Body: Normals, Surface Coefficients, Areas
N(1,:) = n1;    N(2,:) = n2;     N(3,:) = n3;
N(4,:) = -n1;   N(5,:) = -n2;   N(6,:) = -n3;
A(1:N_main) = [a*d a*b b*d a*d a*b b*d]; % [m^2]

% Solar Panels: Normals, Surface Coefficients, Areas
N(7,:) = n1;    N(8,:) = -n1;   N(9,:) = n1;    N(10,:) = -n1;
A(N_main+1:N_main+N_SP) = [c*d c*d c*d c*d]; % [m^2]

% Calculating the position of C.G
r_CG = [-m_main*b/2/(m_main+2*m_SP) 0 0];

% Calculating the position of each surface with respect to C.G
r(1,:) = [0 0 0] - r_CG;  r(2,:) = [-b/2 d/2 0] - r_CG;  r(3,:) = [-b/2 0 a/2] - r_CG;
r(4,:) = [-b 0 0] - r_CG; r(5,:) = [-b/2 -d/2 0] - r_CG; r(6,:) = [-b/2 0 -a/2] - r_CG;
r(7,:) = [0 0 (a+c)/2] - r_CG;   r(8,:)  = [0 0 (a+c)/2] - r_CG;
r(9,:) = [0 0 -(a+c)/2] - r_CG;   r(10,:) = [0 0 -(a+c)/2] - r_CG;


S_B_norm = S_B / norm(S_B);

M_SRP = zeros(3,1);
for k = 1:N_main+N_SP
    if k <= N_main
        rho_s = rho_s_main;     rho_d = rho_d_main;
    else
        rho_s = rho_s_SP;       rho_d = rho_d_SP;
    end
    
    n_k = N(k,:)';
    F_k = - P*A(k)*dot(S_B_norm,n_k) * ( (1-rho_s)*S_B_norm + (2*rho_s*dot(S_B_norm,n_k)+2/3*rho_d)*n_k );
    
    if dot(S_B_norm, n_k) > 0
        r_k = (r(k,:) - r_CG)';
        M_SRP_k = cross(r_k, F_k);
    else
        M_SRP_k = zeros(3,1);
    end
    
    M_SRP = M_SRP + M_SRP_k;
        
end

== matlab function modello_Sabas_friend/Control/M_Detumblling ==
  data: Kp input; M_Detumbling output; w_body input
function M_Detumbling = fcn(Kp, w_body)
M_Detumbling = zeros(3,1);
M_Detumbling(1,1) = Kp(1,1)*w_body(1,1);
M_Detumbling(2,1) = Kp(2,1)*w_body(2,1);
M_Detumbling(3,1) = Kp(3,1)*w_body(3,1);


end

== matlab function modello_Sabas_friend/Disturbances/MATLAB Function4 ==
  data: u input; norm_u output
function norm_u =  fcn(u)

norm_u = norm(u);

== matlab function modello_Sabas_friend/Control/Target Pointing/Target Pointing Algorithm ==
  data: w_b_sensed input; A_e input; Mc output; w_req input; Kp input; Kd input
function Mc  = fcn(w_b_sensed,A_e,w_req,Kp,Kd)

Mx=Kp(1,1)/2*(A_e(2,3)-A_e(3,2))+Kd(1,1)*(w_b_sensed(1)-w_req(1));
My=Kp(2,1)/2*(A_e(3,1)-A_e(1,3))+Kd(2,1)*(w_b_sensed(2)-w_req(2));
Mz=Kp(3,1)/2*(A_e(1,2)-A_e(2,1))+Kd(3,1)*(w_b_sensed(3)-w_req(3));

Mc=[Mx;My;Mz];

== matlab function modello_Sabas_friend/Disturbances/MATLAB Function5 ==
  data: u input; norm_u output
function norm_u =  fcn(u)

norm_u = norm(u);

== matlab function modello_Sabas_friend/Disturbances/MATLAB Function6 ==
  data: u input; norm_u output
function norm_u =  fcn(u)

norm_u = norm(u);

== matlab function modello_Sabas_friend/Disturbances/MATLAB Function7 ==
  data: u input; norm_u output
function norm_u =  fcn(u)

norm_u = norm(u);

== matlab function modello_Sabas_friend/Disturbances/MATLAB Function3 ==
  data: rho input; SC_vars input; kep input; C_D_main input; C_D_SP input; M_Aero output; A_BI input
function M_Aero = Aerodynamic_perturbation(rho, SC_vars, kep, C_D_main, C_D_SP,A_BI)

%% Satellite Characteristics
a = SC_vars(1,1);
b = SC_vars(2,1);
c = SC_vars(3,1);
d = SC_vars(4,1);
m_main = SC_vars(5,1);
m_SP = SC_vars(6,1);

%% Orbit Characteristics
a_orbit  = kep(1);    e  = kep(2);    i = kep(3);
OM = kep(4);    om = kep(5);    th = kep(6);
p = a_orbit*(1-e^2);
R = p / (1+e*cos(th)) * 1e+3; % [m]

%% Aerodynamic Torque

N_main = 6; % # main body surfaces
N_SP = 4; % # solar panel surfaces

N = zeros(N_main+N_SP,3);
A = zeros(N_main+N_SP,1);
r = zeros(N_main+N_SP,3);
n1 = [1 0 0];  n2 = [0 1 0];  n3 = [0 0 1];
% S/C Main Body: Normals, Surface Coefficients, Areas
N(1,:) = n1;    N(2,:) = n2;     N(3,:) = n3;
N(4,:) = -n1;   N(5,:) = -n2;   N(6,:) = -n3;
A(1:N_main) = [a*d a*b b*d a*d a*b b*d]; % [m^2]

% Solar Panels: Normals, Surface Coefficients, Areas
N(7,:) = n1;    N(8,:) = -n1;   N(9,:) = n1;    N(10,:) = -n1;
A(N_main+1:N_main+N_SP) = [c*d c*d c*d c*d]; % [m^2]

% Calculating the position of C.G
r_CG = [-m_main*b/2/(m_main+2*m_SP) 0 0];

% Calculating the position of each surface with respect to C.G
r(1,:) = [0 0 0] - r_CG;  r(2,:) = [-b/2 d/2 0] - r_CG;  r(3,:) = [-b/2 0 a/2] - r_CG;
r(4,:) = [-b 0 0] - r_CG; r(5,:) = [-b/2 -d/2 0] - r_CG; r(6,:) = [-b/2 0 -a/2] - r_CG;
r(7,:) = [0 0 (a+c)/2] - r_CG;   r(8,:)  = [0 0 (a+c)/2] - r_CG;
r(9,:) = [0 0 -(a+c)/2] - r_CG;   r(10,:) = [0 0 -(a+c)/2] - r_CG;


% Earth specifications
w_E = 2*pi/(23*3600 + 56*60 + 4.09); % Earth's angular rate [rad/s]
mu_E = 398600.433; % [km^3/s^2]



% Rotation matrices: Earth-Centered Inertial --> Perifocal   (ECI->PF)
R_om = [cos(om)  sin(om)    0   ;
        -sin(om) cos(om)    0   ;
           0        0       1   ];
       
R_i  = [   1        0       0   ;
           0     cos(i)   sin(i);
           0    -sin(i)   cos(i)];
       
R_OM = [cos(OM)  sin(OM)    0   ;
        -sin(OM) cos(OM)    0   ;
           0        0       1   ];
    
R313 = R_om * R_i * R_OM; % ECI --> PF


R_PF = R * [cos(th), sin(th), 0]';
v_PF = sqrt(mu_E/p) * [-sin(th), (e+cos(th)), 0]';
% PF --> ECI
r_ECI = R313'* R_PF;
v_ECI = R313'* v_PF;


v_rel_I = v_ECI + cross([0 0 w_E]', r_ECI);

v_rel_B = A_BI*v_rel_I; % Relative atmosphere velocity (@body frame)
v_rel_B_unit = v_rel_B / norm(v_rel_B);


M_Aero = zeros(3,1);
for k = 1:N_main+N_SP
    
    if k<=N_main
        C_D = C_D_main;
    else
        C_D = C_D_SP;
    end
    n_k = N(k,:)';
    F_k = - 0.5 * C_D * rho * norm(v_rel_B)^2 * dot(n_k,v_rel_B_unit) * A(k) * v_rel_B_unit;
    
    r_k = (r(k,:) - r_CG)';
    M_drag_k = cross(r_k, F_k);
    
    M_Aero = M_Aero + M_drag_k;
        
end

== matlab function modello_Sabas_friend/Dynamics/Euler Equations ==
  data: w input; M_Control input; I input; w_dot output; M_Disturbance input
function w_dot  = euler_eqs(w, M_Control, I, M_Disturbance)



% Moments of Inertia [kg*m^2]
I1 = I(1,1);
I2 = I(2,2);
I3 = I(3,3);

C1 = (I2-I3)/I1;
C2 = (I3-I1)/I2;
C3 = (I1-I2)/I3;




%% Euler Equations
w_dot = zeros(3,1);
w_dot(1) = C1 * w(2)*w(3) + (M_Control(1) + M_Disturbance(1)) / I1;
w_dot(2) = C2 * w(1)*w(3) + (M_Control(2) + M_Disturbance(2)) / I2;
w_dot(3) = C3 * w(1)*w(2) + (M_Control(3) + M_Disturbance(3)) / I3;

== matlab function modello_Sabas_friend/Dynamics/Moment of Inertia ==
  data: SC_vars input; I output
function I  = Moment_of_Inertia(SC_vars)

%% Satellite Characteristics
a = SC_vars(1,1);
b = SC_vars(2,1);
c = SC_vars(3,1);
d = SC_vars(4,1);
m_main = SC_vars(5,1);
m_SP = SC_vars(6,1);

% Calculating the position of C.G
r_CG = [-m_main*b/2/(m_main+2*m_SP) 0 0];

%% Moments of Inertia [kg*m^2]
I = zeros(3,3);

I(1,1) = m_main*(a^2+d^2)/12 + 2*m_SP*((c^2+d^2)/12+(a/2+c/2)^2);
I(2,2) = m_main*((a^2+b^2)/12+(-b/2-r_CG(1,1))^2) + 2*m_SP*(c^2/12+(a/2+c/2)^2+r_CG(1,1)^2);
I(3,3) = m_main*((b^2+d^2)/12+(-b/2-r_CG(1,1))^2) + 2*m_SP*(d^2/12+r_CG(1,1)^2);

== matlab function modello_Sabas_friend/Kinematics/Euler Angles ==
  data: w input; theta input; theta_dot output
function theta_dot  = euler_angles(w, theta)

theta_dot = zeros(3,1);
%% 321 Euler Angles Set:
theta_dot(1,1) = sin(theta(3,1))*w(2,1)/cos(theta(2,1)) + cos(theta(3,1))*w(3,1)/cos(theta(2,1));
theta_dot(2,1) = cos(theta(3,1))*w(2,1) - sin(theta(3,1))*w(3,1);
theta_dot(3,1) = w(1,1) + sin(theta(3,1))*tan(theta(2,1))*w(2,1) + cos(theta(3,1))*tan(theta(2,1))*w(3,1);

== matlab function modello_Sabas_friend/Kinematics/Direction Cosine Matrix ==
  data: theta input; A_BI output
function A_BI  = DCM(theta)

%% 321 Euler Angles Set:
A_BI = [cos(theta(2,1))*cos(theta(1,1)),cos(theta(2,1))*sin(theta(1,1)),-sin(theta(2,1))
        sin(theta(3,1))*sin(theta(2,1))*cos(theta(1,1))-cos(theta(3,1))*sin(theta(1,1)),sin(theta(3,1))*sin(theta(2,1))*sin(theta(1,1))+cos(theta(3,1))*cos(theta(1,1)),sin(theta(3,1))*cos(theta(2,1))
        cos(theta(3,1))*sin(theta(2,1))*cos(theta(1,1))+sin(theta(3,1))*sin(theta(1,1)),cos(theta(3,1))*sin(theta(2,1))*sin(theta(1,1))-sin(theta(3,1))*cos(theta(1,1)),cos(theta(3,1))*cos(theta(2,1))];

== matlab function modello_Sabas_friend/Kinematics/Transverse Matrices ==
  data: kep input; A_BI input; A_BL output; A_LI output
function [A_BL, A_LI] = fcn(kep, A_BI)
% Orbit elements
i = kep(3);
OM = kep(4);
om = kep(5);
th = kep(6);

% Rotation matrices: Earth-Centered Inertial --> LVLH   (ECI->LVLH)
R_om = [cos(om+th)  sin(om+th)    0   ;
        -sin(om+th) cos(om+th)    0   ;
           0        0       1   ];
       
R_i  = [   1        0       0   ;
           0     cos(i)   sin(i);
           0    -sin(i)   cos(i)];
       
R_OM = [cos(OM)  sin(OM)    0   ;
        -sin(OM) cos(OM)    0   ;
           0        0       1   ];
    
A_LI = R_om * R_i * R_OM;

A_BL = A_BI*A_LI';

== matlab function modello_Sabas_friend/Orbit Propagation/Orbit Propagation ==
  data: kep input; kep_dot output
function kep_dot  = orbit_propagator(kep)

% kep = [a e i om, Om, th]
a  = kep(1);
e  = kep(2);
th = kep(6);

% Calculating orbital angular velocity
mu_e = 398600.433; % [km^3/s^2]
n_e = sqrt(mu_e/a^3);

% Calculating earth angular velocity around the sun
R_s = 149597870.691; % 1AU [km]
mu_s = 132712440017.987;
n_s  = sqrt(mu_s/R_s^3); % [rad/sec]

kep_dot = zeros(6,1);
kep_dot(6,1) = n_e*(1+e*cos(th))^2 / ((1-e^2)^1.5);
kep_dot(5,1) = n_s;

== matlab function modello_Sabas_friend/Orbit Propagation/Sun Direction ==
  data: S_B output; S_I output; A_BI input; dt input
function [S_B, S_I] = sun_direction(A_BI, dt)


R_s = 149597870.691; % 1AU [km]
mu_s = 132712440017.987;
n_s  = sqrt(mu_s/R_s^3);

epsilon = deg2rad(23.45);
% Sun direction w.r.t. S/C ~ Sun direction w.r.t. Earth
S_I = R_s * [cos(n_s*dt), sin(n_s*dt)*cos(epsilon), sin(n_s*dt)*sin(epsilon)]';
S_B = A_BI*S_I;
